simulink subsystem "NOKalmanMeasurement_sim"  (R2024a)
settings: Solver=VariableStepAuto  StartTime=0.0  StopTime=10.0  RelTol=1e-3
undefined symbols (not defined in the file or in its folder): NoiseCov
settings Model: Creator=ruimi  LastModifiedBy=alenachan

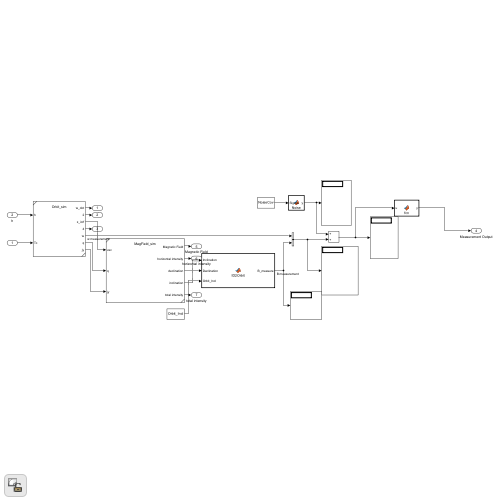
[thumbnail: Simulink's stored preview of the top-level diagram]
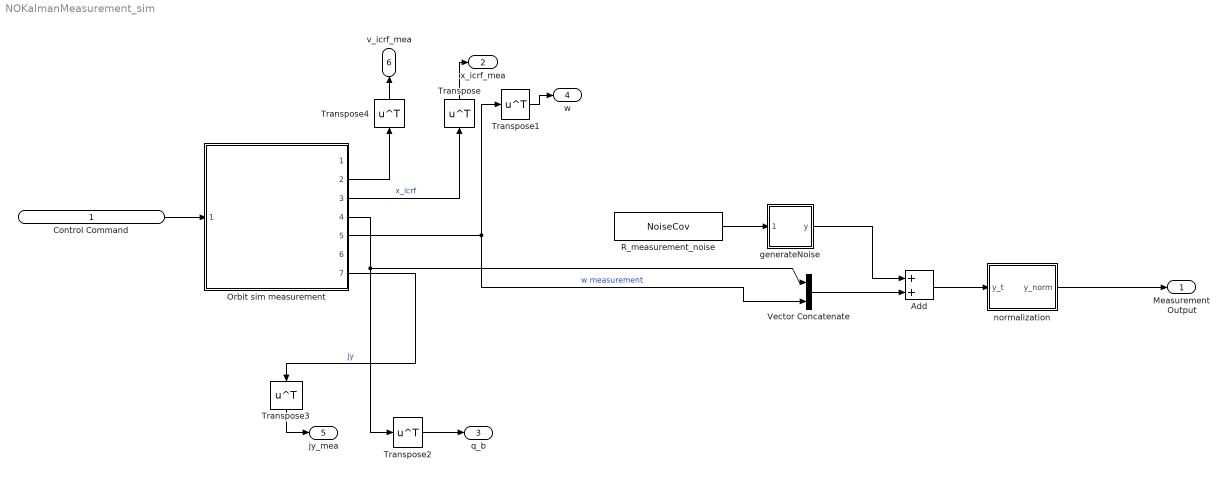
== system NOKalmanMeasurement_sim ==
  Control Command : Inport
  Add : Sum  Priority=7
  Orbit sim measurement : Subsystem  Priority=2  ReferencedSubsystem=Orbit_sim_measurement
  R_measurement_noise : Constant  Value=NoiseCov
  Transpose{,1..4} (5 alike) : Math  Priority=3  Operator=transpose
  Vector Concatenate : Concatenate  Priority=5
  generateNoise : MATLAB Function  Priority=1  TreatAsAtomicUnit=on
  normalization : MATLAB Function  TreatAsAtomicUnit=on
  Measurement Output : Outport
  x_icrf_mea : Outport  Port=2
  q_b : Outport  Port=3
  w : Outport  Port=4
  jy_mea : Outport  Port=5
  v_icrf_mea : Outport  Port=6
  wires:
  Add/1 -> normalization/1(y_t)
  Orbit sim measurement/3 -> Transpose/1  "x_icrf"
  Control Command/1 -> Orbit sim measurement/1
  Orbit sim measurement/7 -> Transpose3/1  "jy"
  Vector Concatenate/1 -> Add/2
  generateNoise/1(y) -> Add/1
  Orbit sim measurement/5 -> Vector Concatenate/2, Transpose1/1  "w measurement"
  R_measurement_noise/1 -> generateNoise/1(Sigma)
  Orbit sim measurement/4 -> Vector Concatenate/1, Transpose2/1
  Transpose/1 -> x_icrf_mea/1
  Transpose1/1 -> w/1
  Transpose2/1 -> q_b/1
  Transpose3/1 -> jy_mea/1
  Orbit sim measurement/2 -> Transpose4/1
  Transpose4/1 -> v_icrf_mea/1
  normalization/1(y_norm) -> Measurement Output/1

== matlab function NOKalmanMeasurement_sim/normalization ==
  data: y_t input; y_norm output
function y_norm = normalizeY(y_t)
y_norm = zeros(7,1);
y_norm(1:4) = y_t(1:4)/norm(y_t(1:4));
y_norm(5:7) = y_t(5:7);

== matlab function NOKalmanMeasurement_sim/generateNoise ==
  data: y output; Sigma input
function y = Noise(Sigma)
secs = mod(mod(now,1)*1000000, 1000);
rng(secs);
mu = [0 0 0 0 0 0 0] ; %mean is zero for noise
%covariance is constant throughout, we take the input
y_temp = mvnrnd(mu,Sigma,1);
y = transpose(y_temp);
end
